simulink model "BPSK_cx_noise_m70"  (Simulink 7.0)
settings: Solver=VariableStepDiscrete  StartTime=0.0  StopTime=sim_t  RelTol=1e-3
undefined symbols (not defined in the file or in its folder): BSTbn, get, PZbn
libraries: commsink2 x3, commdigbbndpm3 x2, commchan3 x1, commrandsrc2 x1
settings Model: Creator=usuario  LastModifiedBy=cocheca
settings DebuggingCC: SaveWithParameterizedLinksMsg=none  SignalResolutionControl=TryResolveAllWithWarning  MultiTaskDSMMsg=warning  MultiTaskCondExecSysMsg=none
settings RTWCC: IncludeERTFirstTime=on
settings GRTTargetCC: TargetFcnLib=ansi_tfl_tmw.mat

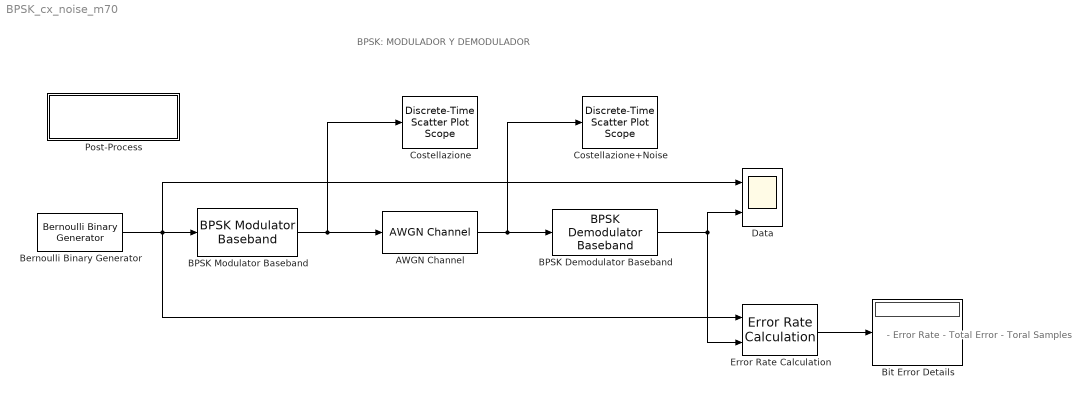
== system BPSK_cx_noise_m70 ==
  note: BPSK: MODULADOR Y DEMODULADOR
  note: - Error Rate
      | - Total Error
      | - Toral Samples
  AWGN Channel : commchan3/AWGN Channel  SystemSampleTime=-1  seed=67  noiseMode="Signal to noise ratio  (SNR)"  EbNodB=20  EsNodB=10  SNRdB=SNRbn  bitsPerSym=1  Ps=1  Tsym=1  variance=1
  BPSK Demodulator Baseband : commdigbbndpm3/BPSK Demodulator Baseband  DialogController=commDDGCreate  DialogControllerArgs=DataTag0  Ph=0  DecType=Hard decision  VarSource=Dialog  Variance=1  outDtype=Inherit via internal rule  derotateFactorWordLen=16
  BPSK Modulator Baseband : commdigbbndpm3/BPSK Modulator Baseband  DialogController=commDDGCreate  DialogControllerArgs=DataTag1  SystemSampleTime=-1  Ph=0  outDtype=double  outWordLen=16  outUDDataType=sfix(16)  outFracLenMode=Best precision  outFracLen=15
  Bernoulli Binary Generator : commrandsrc2/Bernoulli Binary Generator  DialogController=commDDGCreate  DialogControllerArgs=DataTag2  SystemSampleTime=-1  P=PZbn  seed=51  Ts=BSTbn  frameBased=off  sampPerFrame=1  orient=off  outDataType=double
  Bit Error Details : Display
  "Costellazione " : commsink2/Discrete-Time Scatter Plot Scope  Tag=ScatterPlot  SystemSampleTime=-1  sampPerSymb=1  offsetEye=0  numTraces=40  numNewFrames=10  LineMarkers=x  LineColors=k  fading=on  render=on  AxisGrid=on  xMin=-3.3  xMax=3.315  yMin=-3.3  yMax=3.315  inphaseLabel=In-phase Amplitude  quadratureLabel=Quadrature Amplitude  openScopeAtSimStart=on  FrameNumber=off  FigPos=get(0,'defaultfigureposition');  figTitle=Scatter Plot  numLinesMax=8  block_type_=scatter
  Costellazione+Noise : commsink2/Discrete-Time Scatter Plot Scope  Tag=ScatterPlot  SystemSampleTime=-1  sampPerSymb=1  offsetEye=0  numTraces=40  numNewFrames=10  LineMarkers=x  LineColors=k  fading=on  render=on  AxisGrid=on  xMin=-3.3  xMax=3.315  yMin=-3.3  yMax=3.315  inphaseLabel=In-phase Amplitude  quadratureLabel=Quadrature Amplitude  openScopeAtSimStart=on  FrameNumber=off  FigPos=get(0,'defaultfigureposition');  figTitle=Scatter Plot  numLinesMax=8  block_type_=scatter
  Data : Scope  NumInputPorts=2
      settings: YMin=-0.5~-0.5  YMax=1.5~1.5  SaveName=ScopeData3
  Error Rate Calculation : commsink2/Error Rate Calculation  N=0  st_delay=0  cp_mode=Entire frame  subframe=[]  PMode=Port  WsName=ErrorVec  RsMode2=off  stop=off  numErr=100  maxBits=1e6
  Post-Process : Subsystem  mask{sim_t=1000, BSTbn=5, SNRbn=0}
      mask prompts: sim_t "Sim Time [100]"; BSTbn "Source Sample Time"; SNRbn "SNR"
      mask init:
      | %sim_t = 100; %simulation time
      | %BSTf = 5; % source sample time
      | PZbn = .4; % probability of zero
      | 
      | %STf = 1/100; % sample time
      | %A1f = 1; % amplitude sine 1 - mod.
      | %A2f = 1; % amplitude sine 2 - mod.
      | %F1f = 2*pi*8; % Freg Sine 1
      | %F2f = 2*pi*12; % Freg Sine 2
      | 
      | 
      | % Sample Time Source Configure
      | switch BSTbn
      |     case 1
      |         BSTbn = 1;
      |     case 2
      |         BSTbn = 5;
      |     case 3
      |         BSTbn = 10;      
      | end
      | 
      | % switch SNRbn
      | %     case 1
      | %         SNRbn = -10;
      | %     case 2
      | %         SNRbn = -5;
      | %     case 3
      | %         SNRbn = 0;
      | %     case 4
      | %         SNRbn = 5;
      | %     case 5
      | %         SNRbn = 10;        
      | %     case 6
      | %         SNRbn = 20;        
      | % end
      | 
      | switch sim_t
      |     case 1
      |         sim_t = 50;
      |     case 2
      |         sim_t = 100;
      |     case 3
      |         sim_t = 250;
      |     case 4
      |         sim_t = 500;
      |     case 5
      |         sim_t = 1000;        
      | end
      | 
      | 
      | assignin('base','sim_t', sim_t );
      | assignin('base','BSTbn', BSTbn );
      | assignin('base','PZbn', PZbn );
      | assignin('base','SNRbn', SNRbn );
      mask StyleString: popup(50|100|250|500|1000),popup(1|5|10),edit
      mask Display: disp('Sim Parameters')
  wires:
  Bernoulli Binary Generator/1 -> Data/1, Error Rate Calculation/1, BPSK Modulator Baseband/1
  BPSK Modulator Baseband/1 -> AWGN Channel/1, "Costellazione "/1
  AWGN Channel/1 -> BPSK Demodulator Baseband/1, Costellazione+Noise/1
  BPSK Demodulator Baseband/1 -> Error Rate Calculation/2, Data/2
  Error Rate Calculation/1 -> Bit Error Details/1

== system BPSK_cx_noise_m70/Post-Process ==
